simulink library "ModG_Transformaciones"  (R2018a)
settings: Solver=VariableStepAuto  StartTime=0.0  StopTime=10.0  RelTol=1e-3
libraries: $bdroot x6
settings Model: Creator=Guillermo  LastModifiedBy=Lisandro Cocca

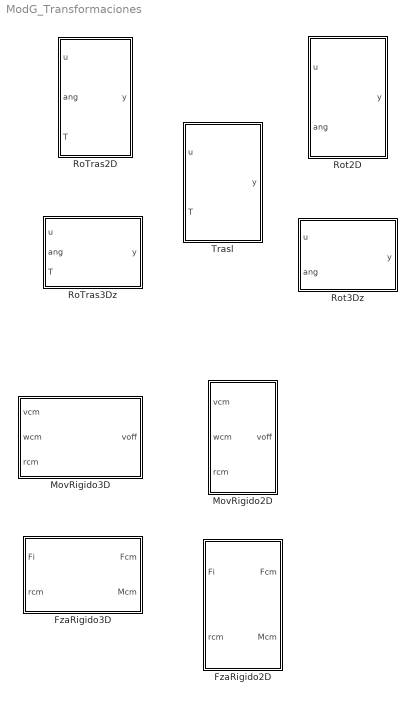
== system ModG_Transformaciones ==
  FzaRigido2D : Subsystem
  FzaRigido3D : Subsystem
  MovRigido2D : Subsystem
  MovRigido3D : Subsystem
  RoTras2D : Subsystem
  RoTras3Dz : Subsystem
  Rot2D : Subsystem
  Rot3Dz : Subsystem
  Trasl : Subsystem

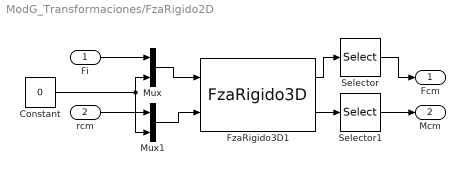
== system ModG_Transformaciones/FzaRigido2D ==
  Fi : Inport  PortDimensions=2
  rcm : Inport  Port=2  PortDimensions=2
  Constant : Constant  Value=0
  FzaRigido3D1 : $bdroot/FzaRigido3D
  Mux : Mux  Inputs=2
  Mux1 : Mux  Inputs=2
  Selector : Selector  InputPortWidth=3  IndexOptions=Index vector (dialog)  Indices=[1 2]  OutputSizes=1
  Selector1 : Selector  InputPortWidth=3  IndexOptions=Index vector (dialog)  Indices=3  OutputSizes=1
  Fcm : Outport  PortDimensions=2
  Mcm : Outport  Port=2  PortDimensions=1
  wires:
  Selector/1 -> Fcm/1
  Constant/1 -> Mux1/2, Mux/2
  FzaRigido3D1/1 -> Selector/1
  FzaRigido3D1/2 -> Selector1/1
  Mux/1 -> FzaRigido3D1/1
  Mux1/1 -> FzaRigido3D1/2
  Fi/1 -> Mux/1
  rcm/1 -> Mux1/1
  Selector1/1 -> Mcm/1

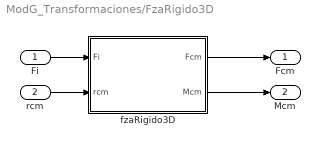
== system ModG_Transformaciones/FzaRigido3D ==
  Fi : Inport  PortDimensions=3
  rcm : Inport  Port=2  PortDimensions=3
  fzaRigido3D : MATLAB Function  TreatAsAtomicUnit=on
  Fcm : Outport  PortDimensions=3
  Mcm : Outport  Port=2  PortDimensions=3
  wires:
  fzaRigido3D/2(Mcm) -> Mcm/1
  Fi/1 -> fzaRigido3D/1(Fi)
  fzaRigido3D/1(Fcm) -> Fcm/1
  rcm/1 -> fzaRigido3D/2(rcm)

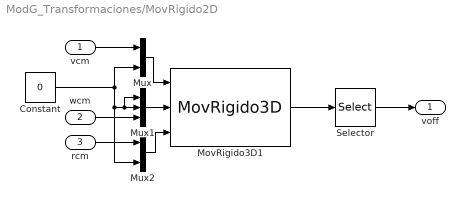
== system ModG_Transformaciones/MovRigido2D ==
  vcm : Inport  PortDimensions=2
  wcm : Inport  Port=2  PortDimensions=1
  rcm : Inport  Port=3  PortDimensions=2
  Constant : Constant  Value=0
  MovRigido3D1 : $bdroot/MovRigido3D
  Mux : Mux  Inputs=2
  Mux1 : Mux  Inputs=3
  Mux2 : Mux  Inputs=2
  Selector : Selector  InputPortWidth=3  IndexOptions=Index vector (dialog)  Indices=[1 2]  OutputSizes=1
  voff : Outport
  wires:
  Constant/1 -> Mux/2, Mux1/1, Mux1/2, Mux2/2
  MovRigido3D1/1 -> Selector/1
  Selector/1 -> voff/1
  Mux2/1 -> MovRigido3D1/3
  rcm/1 -> Mux2/1
  wcm/1 -> Mux1/3
  Mux/1 -> MovRigido3D1/1
  vcm/1 -> Mux/1
  Mux1/1 -> MovRigido3D1/2

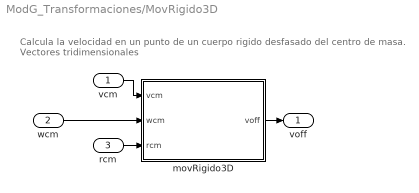
== system ModG_Transformaciones/MovRigido3D ==
  note: Calcula la velocidad en un punto de un cuerpo rigido desfasado del centro de masa.
      | Vectores tridimensionales
  vcm : Inport  PortDimensions=3
  wcm : Inport  Port=2  PortDimensions=3
  rcm : Inport  Port=3  PortDimensions=3
  movRigido3D : MATLAB Function  TreatAsAtomicUnit=on
  voff : Outport  PortDimensions=3
  wires:
  vcm/1 -> movRigido3D/1(vcm)
  wcm/1 -> movRigido3D/2(wcm)
  movRigido3D/1(voff) -> voff/1
  rcm/1 -> movRigido3D/3(rcm)

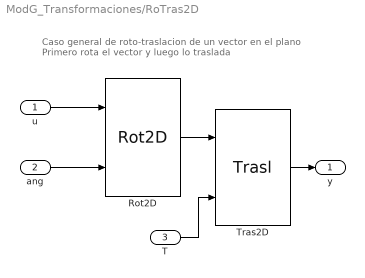
== system ModG_Transformaciones/RoTras2D ==
  note: Caso general de roto-traslacion de un vector en el plano
      | Primero rota el vector y luego lo traslada
  u : Inport  PortDimensions=2
  ang : Inport  Port=2  PortDimensions=1
  T : Inport  Port=3  PortDimensions=2
  Rot2D : $bdroot/Rot2D
  Tras2D : $bdroot/Trasl
  y : Outport  PortDimensions=2
  wires:
  ang/1 -> Rot2D/2
  T/1 -> Tras2D/2
  Tras2D/1 -> y/1
  u/1 -> Rot2D/1
  Rot2D/1 -> Tras2D/1

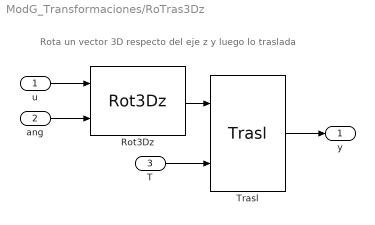
== system ModG_Transformaciones/RoTras3Dz ==
  note: Rota un vector 3D respecto del eje z y luego lo traslada
  u : Inport  PortDimensions=3
  ang : Inport  Port=2  PortDimensions=1
  T : Inport  Port=3  PortDimensions=3
  Rot3Dz : $bdroot/Rot3Dz
  Trasl : $bdroot/Trasl
  y : Outport  PortDimensions=3
  wires:
  u/1 -> Rot3Dz/1
  ang/1 -> Rot3Dz/2
  Rot3Dz/1 -> Trasl/1
  T/1 -> Trasl/2
  Trasl/1 -> y/1

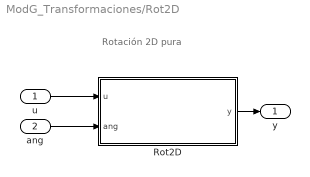
== system ModG_Transformaciones/Rot2D ==
  note: Rotación 2D pura
  u : Inport  PortDimensions=2
  ang : Inport  Port=2  PortDimensions=1
  "Rot2D " : MATLAB Function  TreatAsAtomicUnit=on
  y : Outport
  wires:
  u/1 -> "Rot2D "/1(u)
  "Rot2D "/1(y) -> y/1
  ang/1 -> "Rot2D "/2(ang)

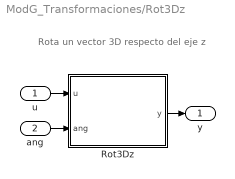
== system ModG_Transformaciones/Rot3Dz ==
  note: Rota un vector 3D respecto del eje z
  u : Inport  PortDimensions=3
  ang : Inport  Port=2  PortDimensions=1
  Rot3Dz : MATLAB Function  TreatAsAtomicUnit=on
  y : Outport  PortDimensions=3
  wires:
  u/1 -> Rot3Dz/1(u)
  Rot3Dz/1(y) -> y/1
  ang/1 -> Rot3Dz/2(ang)

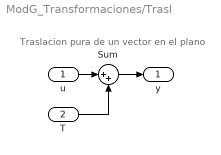
== system ModG_Transformaciones/Trasl ==
  note: Traslacion pura de un vector en el plano
  u : Inport
  T : Inport  Port=2
  Sum : Sum  Inputs=|++
  y : Outport
  wires:
  u/1 -> Sum/1
  T/1 -> Sum/2
  Sum/1 -> y/1

== matlab function ModG_Transformaciones/MovRigido3D/movRigido3D ==
  data: vcm input; voff output; wcm input; rcm input
function voff = movRigido3D(vcm, wcm, rcm)
% Calcula la velocidad en un punto de un cuerpo rígido a partir de las
% velocidades del centro de masa y posicion relativa. Vectores 3D!!

voff = vcm + cross(wcm,rcm);

== matlab function ModG_Transformaciones/Rot3Dz/Rot3Dz ==
  data: u input; y output; ang input
function y = Rot3Dz(u,ang)
% Rota un vector tridimensional respecto del eje z
y = [cos(ang) -sin(ang) 0; sin(ang) cos(ang) 0; 0 0 1]*u;

== matlab function ModG_Transformaciones/Rot2D/Rot2D  ==
  data: u input; y output; ang input
function y = Rot2D(u, ang)
% Rota y luego traslada un vector 2D
%   u: vector de entradas
%   ang: angulo de giro
%   T:  vector de traslacion
y = [cos(ang) -sin(ang); sin(ang) cos(ang)]*u;

== matlab function ModG_Transformaciones/FzaRigido3D/fzaRigido3D ==
  data: Fi input; Fcm output; rcm input; Mcm output
function [Fcm,Mcm] = fzaRigido3D(Fi, rcm)
% Calcula las fuerzas y momentos en el centro de masa de un cuerpo rigido
% como efectos de una fuerza en un punto desfasado del centro masa.
Fcm = Fi;
Mcm = cross(rcm,Fi);
